simulink model "LAB2_2_DirectDigitalDesign_2024b"  (R2024b)
settings: Solver=FixedStepDiscrete  StartTime=0.0  StopTime=5  FixedStep=T  RelTol=1e-3
values from neighbouring files (symbols this model uses):
  gamma_o = [gamma(2)-L*gamma(1), (phi22-L*phi12)*L+phi21-L*phi11]    [LAB2_2_DirectDigitalDesign.m]
  Ho = [0;1]    [LAB2_2_DirectDigitalDesign.m]
  Jo = [0 1; 0 L]    [LAB2_2_DirectDigitalDesign.m]
  K = Ke(2:3)    [LAB2_2_DirectDigitalDesign.m]
  Ki = Ke(1)    [LAB2_2_DirectDigitalDesign.m]
  Nr = Nu + K * Nx    [LAB2_2_DirectDigitalDesign.m]
  phi_o = lambda_o_dt    [LAB2_2_DirectDigitalDesign.m]
  step_amplitude = 50    [LAB2_2_DirectDigitalDesign.m]
  T = 0.05    [LAB2_2_DirectDigitalDesign.m]
undefined symbols (not defined in the file or in its folder): den_Hi, DiscIntNeverNeededParam, mot, National_Instruments, num_Hi, PCI, pulse2deg, sens
libraries: sldrtlib x3
settings Model: SimulationMode=external  ExtModeTrigDuration=100001  Creator=delpratogi  LastModifiedBy=delpratogi
settings HardwareCC: ProdBitPerLong=64  ProdHWDeviceType=Intel->x86-64 (Linux 64)
settings RTWCC: Description=Simulink Desktop Real-Time  SystemTargetFile=sldrt.tlc  TemplateMakefile=sldrt.tmf  RTWCompilerOptimization=on
settings CodeAppCC: MaxIdLength=95
settings SimulinkDesktopRealTimeCC: TargetLibSuffix=_sldrt.a  TargetPreCompLibLocation=C:\Program Files\MATLAB\R2024b\toolbox\sldrt\lib\win64  ParMdlRefBuildCompliant=on  SupportVariableSizeSignals=off

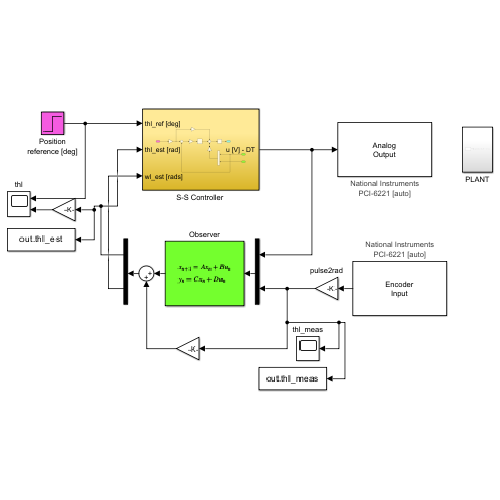
[thumbnail: Simulink's stored preview of the top-level diagram]
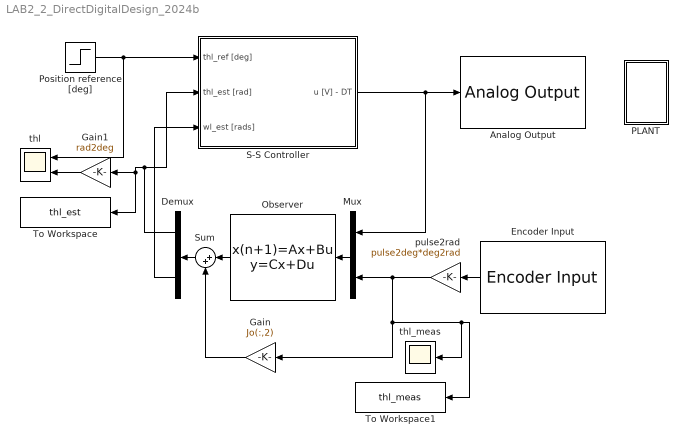
== system LAB2_2_DirectDigitalDesign_2024b ==
  Analog Output : sldrtlib/Analog Output  SampleTime=T  MaxMissedTicks=10  ShowMissedTicks=off  YieldWhenWaiting=off  DrvName=National_Instruments/PCI-6221  DrvAddress=4294967295  DrvOptions=[0 0 0 2 0]  Channels=1  RangeMode=1  VoltRange=1  InitialValue=0  FinalValue=0
      settings: AttributesFormatString=National Instruments\nPCI-6221 [auto]
  Demux : Demux  Outputs=2
  Encoder Input : sldrtlib/Encoder Input  SampleTime=T  MaxMissedTicks=10  ShowMissedTicks=off  YieldWhenWaiting=off  DrvName=National_Instruments/PCI-6221  DrvAddress=4294967295  DrvOptions=[0 0 0 2 0]  Channels=1  QuadMode=3  IndexPulse=1  InputFilter=Inf  DataType=1
      settings: AttributesFormatString=National Instruments\nPCI-6221 [auto]
  Gain : Gain  Gain=Jo(:,2)
  Gain1 : Gain  Gain=rad2deg
  Mux : Mux  Inputs=2
  Observer : DiscreteStateSpace  A=phi_o  B=gamma_o  C=Ho  D=zeros(2,2)  SampleTime=T
  PLANT : Subsystem
  Position reference [deg] : Step  After=step_amplitude  SampleTime=T  ZeroCross=off
  "S-S Controller " : Subsystem
  Sum : Sum  Inputs=|++
  To Workspace : ToWorkspace  VariableName=thl_est  SaveFormat=Structure With Time  SampleTime=T
  To Workspace1 : ToWorkspace  VariableName=thl_meas  SaveFormat=Structure With Time  SampleTime=T
  pulse2rad : Gain  Gain=pulse2deg*deg2rad
  thl : Scope  NumInputPorts=2
  thl_meas : Scope
  wires:
  Demux/2 -> "S-S Controller "/3(wl_est [rads])
  "S-S Controller "/1("u [V] - DT ") -> Analog Output/1, Mux/1
  Demux/1 -> "S-S Controller "/2(thl_est [rad]), To Workspace/1, Gain1/1
  Position reference [deg]/1 -> thl/1, "S-S Controller "/1(thl_ref [deg])
  Mux/1 -> Observer/1
  Encoder Input/1 -> pulse2rad/1
  pulse2rad/1 -> Gain/1, thl_meas/1, To Workspace1/1, Mux/2
  Sum/1 -> Demux/1
  Observer/1 -> Sum/1
  Gain/1 -> Sum/2
  Gain1/1 -> thl/2

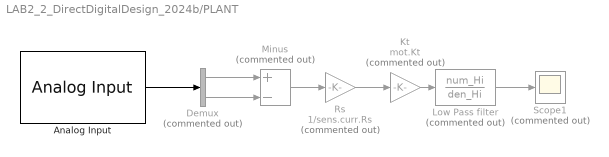
== system LAB2_2_DirectDigitalDesign_2024b/PLANT ==
  Analog Input : sldrtlib/Analog Input  SampleTime=T  MaxMissedTicks=10  ShowMissedTicks=off  YieldWhenWaiting=off  DrvName=National_Instruments/PCI-6221  DrvAddress=4294967295  DrvOptions=[0 0 0 2 0]  Channels=[1,2]  RangeMode=1  VoltRange=1  DataType=1
      settings: AttributesFormatString=National Instruments\nPCI-6221 [auto]
  Demux : Demux  Commented=on  Outputs=2
  Kt : Gain  Commented=on  Gain=mot.Kt
  Low Pass filter : TransferFcn  Commented=on  Numerator=num_Hi  Denominator=den_Hi
  Minus : Sum  Commented=on  Inputs=+-
  Rs : Gain  Commented=on  Gain=1/sens.curr.Rs
  Scope1 : Scope  Commented=on
  wires:
  Low Pass filter/1 -> Scope1/1
  Demux/1 -> Minus/1
  Minus/1 -> Rs/1
  Analog Input/1 -> Demux/1
  Kt/1 -> Low Pass filter/1
  Demux/2 -> Minus/2
  Rs/1 -> Kt/1

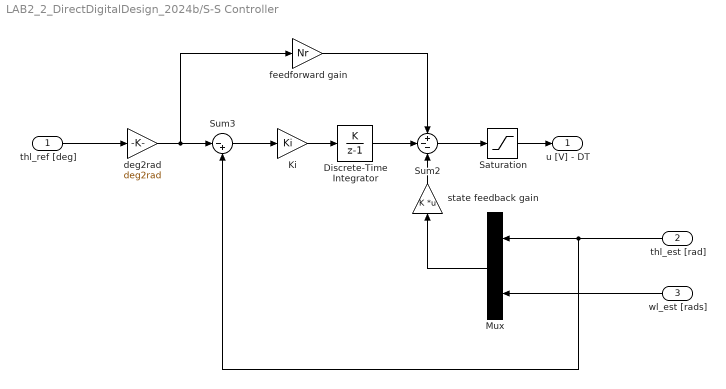
== system LAB2_2_DirectDigitalDesign_2024b/S-S Controller  ==
  thl_ref [deg] : Inport
  thl_est [rad] : Inport  Port=2
  wl_est [rads] : Inport  Port=3
  " feedforward gain" : Gain  Gain=Nr
  Discrete-Time Integrator : DiscreteIntegrator  IntegratorMethod=Accumulation: Forward Euler  SampleTime=T  ICPrevOutput=DiscIntNeverNeededParam  ICPrevScaledInput=DiscIntNeverNeededParam
  Ki : Gain  Gain=Ki
  Mux : Mux  Inputs=2
  Saturation : Saturate  UpperLimit=10  LowerLimit=-10  ZeroCross=off
  Sum2 : Sum  Inputs=+--
  Sum3 : Sum  Inputs=|-+
  deg2rad : Gain  Gain=deg2rad
  state feedback gain : Gain  Gain=K  Multiplication=Matrix(K*u)
  "u [V] - DT " : Outport
  wires:
  Mux/1 -> state feedback gain/1
  Ki/1 -> Discrete-Time Integrator/1
  deg2rad/1 -> " feedforward gain"/1, Sum3/1
  Sum2/1 -> Saturation/1
  Saturation/1 -> "u [V] - DT "/1
  thl_est [rad]/1 -> Sum3/2, Mux/1
  Sum3/1 -> Ki/1
  state feedback gain/1 -> Sum2/3
  " feedforward gain"/1 -> Sum2/1
  thl_ref [deg]/1 -> deg2rad/1
  wl_est [rads]/1 -> Mux/2
  Discrete-Time Integrator/1 -> Sum2/2
